simulink model "task_I_mod"  (R2018a)
settings: Solver=ode4  StartTime=0.0  StopTime=10.0  FixedStep=0.01  RelTol=1e-3  EnableMultiTasking=on
values from neighbouring files (symbols this model uses):
  Ln = 1; sim('task_A_mod')    [task_A_scr.m]    (also in task_C_scr.m = 10; sim('task_C_mod'); task_D_scr.m = 10; sim('task_D_mod'); task_E_scr.m = 10; sim('task_E_mod',5); task_F_scr.m = 10; sim('task_E_mod',20))
  nois = 1; sim('task_H_mod')    [task_H_scr.m]    (also in task_I_scr.m = 1; sim('task_I_mod'); task_J_scr.m = 1; sim('task_J_mod'))
libraries: simulink x1
settings Model: Creator=Yurii  LastModifiedBy=Master
settings DataIOCC: LimitDataPoints=on  SaveFormat=Array
settings OptimizationCC: LifeSpan=inf
settings DebuggingCC: UnderspecifiedInitializationDetection=Classic  MergeDetectMultiDrivingBlocksExec=none  SolverPrmCheckMsg=warning  SFUnexpectedBacktrackingDiag=warning  SFNoUnconditionalDefaultTransitionDiag=warning  SFExecutionAtInitializationDiag=none
settings HardwareCC: ProdBitPerPointer=32  ProdBitPerSizeT=32  ProdBitPerPtrDiffT=32  ProdLargestAtomicFloat=None  ProdIntDivRoundTo=Undefined  ProdEndianess=Unspecified  ProdWordSize=32  ProdHWDeviceType=32-bit Generic
settings ModelReferenceCC: PropagateSignalLabelsOutOfModel=off
settings CodeAppCC: StateflowObjectComments=on
settings GRTTargetCC: TargetLangStandard=C89/C90 (ANSI)  GeneratePreprocessorConditionals=Disable all
settings ConfigComp: CovMetricSettings=dw  CovHtmlReporting=on  CovSaveCumulativeToWorkspaceVar=on  CovSaveSingleToWorkspaceVar=on  CovExternalEMLEnable=off

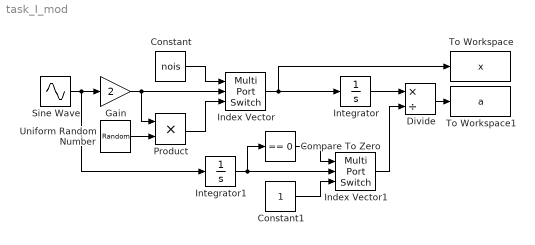
== system task_I_mod ==
  Compare To Zero : simulink/Logic and Bit Operations/Compare To Zero  relop===  OutDataTypeStr=boolean
  Constant : Constant  Value=nois
  Constant1 : Constant
  Divide : Product  Inputs=*/
  Gain : Gain  Gain=2
  Index Vector : MultiPortSwitch  DataPortOrder=Zero-based contiguous  Inputs=2  zeroidx=on
  Index Vector1 : MultiPortSwitch  DataPortOrder=Zero-based contiguous  Inputs=2  zeroidx=on
  Integrator : Integrator
  Integrator1 : Integrator
  Product : Product
  Sine Wave : Sin  SampleTime=0
  To Workspace : ToWorkspace  VariableName=x  SaveFormat=Timeseries  SampleTime=-1
  To Workspace1 : ToWorkspace  VariableName=a  SaveFormat=Timeseries  SampleTime=-1
  Uniform Random Number : UniformRandomNumber  Minimum=1-Ln/100  Maximum=1+Ln/100  SampleTime=0.0
  wires:
  Sine Wave/1 -> Integrator1/1, Gain/1
  Gain/1 -> Index Vector/2, Product/1
  Uniform Random Number/1 -> Product/2
  Integrator1/1 -> Compare To Zero/1, Index Vector1/2
  Constant/1 -> Index Vector/1
  Product/1 -> Index Vector/3
  Index Vector/1 -> To Workspace/1, Integrator/1
  Integrator/1 -> Divide/1
  Compare To Zero/1 -> Index Vector1/1
  Index Vector1/1 -> Divide/2
  Constant1/1 -> Index Vector1/3
  Divide/1 -> To Workspace1/1
